simulink model "sogi_discrete_comparison"  (R2026a)
settings: Solver=FixedStepDiscrete  StopTime=1  FixedStep=double(Cal_SOGI_Ts_s_f32)
PostLoadFcn:
  | addpath(fileparts(get_param('sogi_discrete_comparison','FileName'))); sogi_refresh_parameter_panels('sogi_discrete_comparison');
InitFcn:
  | sogi_check_parameter_binding('sogi_discrete_comparison',false);
StartFcn:
  | sogi_check_parameter_binding('sogi_discrete_comparison',true,true);
values from neighbouring files (symbols this model uses):
  Cal_SOGI_BEA11_f32 = 0.978032291    [sogi_parameters.sldd]
  Cal_SOGI_BEA12_f32 = -0.0153628942    [sogi_parameters.sldd]
  Cal_SOGI_BEA21_f32 = 0.0153628942    [sogi_parameters.sldd]
  Cal_SOGI_BEA22_f32 = 0.999758661    [sogi_parameters.sldd]
  Cal_SOGI_BEB11_f32 = 0.0217264127    [sogi_parameters.sldd]
  Cal_SOGI_BEB21_f32 = 0.000341277686    [sogi_parameters.sldd]
  Cal_SOGI_BEC11_f32 = 0.978032291    [sogi_parameters.sldd]
  Cal_SOGI_BEC12_f32 = -0.0153628942    [sogi_parameters.sldd]
  Cal_SOGI_BEC21_f32 = 0.0153628942    [sogi_parameters.sldd]
  Cal_SOGI_BEC22_f32 = 0.999758661    [sogi_parameters.sldd]
  Cal_SOGI_BED11_f32 = 0.0217264127    [sogi_parameters.sldd]
  Cal_SOGI_BED21_f32 = 0.000341277686    [sogi_parameters.sldd]
  Cal_SOGI_Ts_s_f32 = 5.0E-5    [sogi_parameters.sldd]
  Cal_SOGI_TustinA11_f32 = 0.977908969    [sogi_parameters.sldd]
  Cal_SOGI_TustinA12_f32 = -0.0155344605    [sogi_parameters.sldd]
  Cal_SOGI_TustinA21_f32 = 0.0155344605    [sogi_parameters.sldd]
  Cal_SOGI_TustinA22_f32 = 0.999878    [sogi_parameters.sldd]
  Cal_SOGI_TustinB11_f32 = 0.0219690446    [sogi_parameters.sldd]
  Cal_SOGI_TustinB21_f32 = 0.00017254446    [sogi_parameters.sldd]
  Cal_SOGI_TustinC11_f32 = 0.988954484    [sogi_parameters.sldd]
  Cal_SOGI_TustinC12_f32 = -0.00776723027    [sogi_parameters.sldd]
  Cal_SOGI_TustinC21_f32 = 0.00776723027    [sogi_parameters.sldd]
  Cal_SOGI_TustinC22_f32 = 0.999939    [sogi_parameters.sldd]
  Cal_SOGI_TustinD11_f32 = 0.0109845223    [sogi_parameters.sldd]
  Cal_SOGI_TustinD21_f32 = 8.627223E-5    [sogi_parameters.sldd]
  Cal_SOGI_ZOHA11_f32 = 0.977908969    [sogi_parameters.sldd]
  Cal_SOGI_ZOHA12_f32 = -0.0155341374    [sogi_parameters.sldd]
  Cal_SOGI_ZOHA21_f32 = 0.0155341374    [sogi_parameters.sldd]
  Cal_SOGI_ZOHA22_f32 = 0.999877512    [sogi_parameters.sldd]
  Cal_SOGI_ZOHB11_f32 = 0.0219685864    [sogi_parameters.sldd]
  Cal_SOGI_ZOHB21_f32 = 0.000173183245    [sogi_parameters.sldd]
  Cal_SOGI_ZOHC11_f32 = 1.0    [sogi_parameters.sldd]
  Cal_SOGI_ZOHC12_f32 = 0.0    [sogi_parameters.sldd]
  Cal_SOGI_ZOHC21_f32 = 0.0    [sogi_parameters.sldd]
  Cal_SOGI_ZOHC22_f32 = 1.0    [sogi_parameters.sldd]
  Cal_SOGI_ZOHD11_f32 = 0.0    [sogi_parameters.sldd]
  Cal_SOGI_ZOHD21_f32 = 0.0    [sogi_parameters.sldd]
settings Model: DataDictionary=sogi_parameters.sldd  EnableAccessToBaseWorkspace=off  Creator=ASUS  LastModifiedBy=ASUS

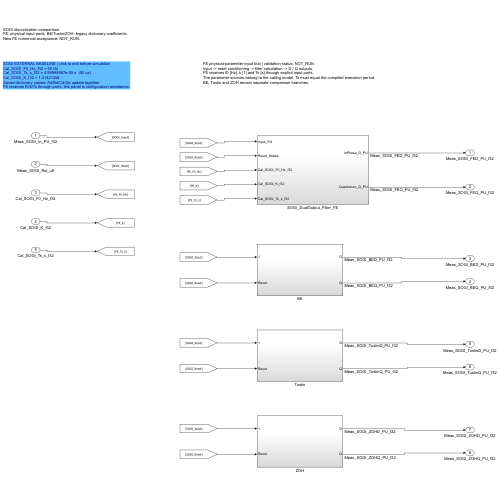
[thumbnail: Simulink's stored preview of the top-level diagram]
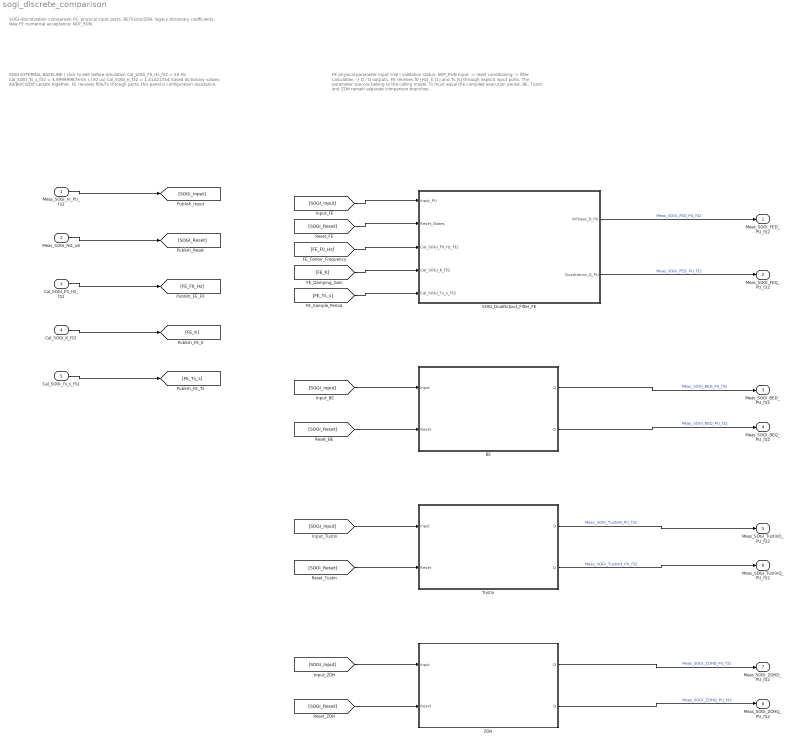
== system sogi_discrete_comparison ==
  note: SOGI discretization comparison
      | FE: physical input ports. BE/Tustin/ZOH: legacy dictionary coefficients.
      | New FE numerical acceptance: NOT_RUN.
  note: SOGI EXTERNAL BASELINE | click to edit before simulation
      | Cal_SOGI_F0_Hz_f32 = 50 Hz
      | Cal_SOGI_Ts_s_f32 = 4.99999987e-05 s  (50 us)
      | Cal_SOGI_K_f32 = 1.41421354
      | Saved dictionary values; Ad/Bd/Cd/Dd update together.
      | FE receives f0/k/Ts through ports; this panel is configuration assistance.
  note: FE physical-parameter input trial | validation status: NOT_RUN
      | Input -> reset conditioning -> filter calculation -> D / Q outputs.
      | FE receives f0 [Hz], k [1] and Ts [s] through explicit input ports.
      | The parameter sources belong to the calling model. Ts must equal the compiled execution period.
      | BE, Tustin and ZOH remain separate comparison branches.
  Meas_SOGI_In_PU_f32 : Inport  OutDataTypeStr=single  SampleTime=double(Cal_SOGI_Ts_s_f32)
  Meas_SOGI_Rst_u8 : Inport  Port=2  OutDataTypeStr=uint8  SampleTime=double(Cal_SOGI_Ts_s_f32)
  Cal_SOGI_F0_Hz_f32 : Inport  Port=3  OutDataTypeStr=single  SampleTime=double(Cal_SOGI_Ts_s_f32)
  Cal_SOGI_K_f32 : Inport  Port=4  OutDataTypeStr=single  SampleTime=double(Cal_SOGI_Ts_s_f32)
  Cal_SOGI_Ts_s_f32 : Inport  Port=5  OutDataTypeStr=single  SampleTime=double(Cal_SOGI_Ts_s_f32)
  BE : Subsystem
  SOGI_DualOutput_Filter_FE : Subsystem  Tag=SOGI_METHOD_FE
  Tustin : Subsystem
  ZOH : Subsystem
  Meas_SOGI_FED_PU_f32 : Outport  OutDataTypeStr=single
  Meas_SOGI_FEQ_PU_f32 : Outport  Port=2  OutDataTypeStr=single
  Meas_SOGI_BED_PU_f32 : Outport  Port=3  OutDataTypeStr=single
  Meas_SOGI_BEQ_PU_f32 : Outport  Port=4  OutDataTypeStr=single
  Meas_SOGI_TustinD_PU_f32 : Outport  Port=5  OutDataTypeStr=single
  Meas_SOGI_TustinQ_PU_f32 : Outport  Port=6  OutDataTypeStr=single
  Meas_SOGI_ZOHD_PU_f32 : Outport  Port=7  OutDataTypeStr=single
  Meas_SOGI_ZOHQ_PU_f32 : Outport  Port=8  OutDataTypeStr=single
  wires:
  [SOGI_Reset] -> ZOH/2(Reset)
  [SOGI_Input] -> ZOH/1(Input)
  [SOGI_Reset] -> Tustin/2(Reset)
  [SOGI_Input] -> Tustin/1(Input)
  [SOGI_Reset] -> BE/2(Reset)
  [SOGI_Input] -> BE/1(Input)
  [SOGI_Reset] -> SOGI_DualOutput_Filter_FE/2(Reset_States)
  [SOGI_Input] -> SOGI_DualOutput_Filter_FE/1(Input_PU)
  ZOH/2(Q) -> Meas_SOGI_ZOHQ_PU_f32/1  "Meas_SOGI_ZOHQ_PU_f32"
  ZOH/1(D) -> Meas_SOGI_ZOHD_PU_f32/1  "Meas_SOGI_ZOHD_PU_f32"
  Tustin/2(Q) -> Meas_SOGI_TustinQ_PU_f32/1  "Meas_SOGI_TustinQ_PU_f32"
  Tustin/1(D) -> Meas_SOGI_TustinD_PU_f32/1  "Meas_SOGI_TustinD_PU_f32"
  BE/2(Q) -> Meas_SOGI_BEQ_PU_f32/1  "Meas_SOGI_BEQ_PU_f32"
  BE/1(D) -> Meas_SOGI_BED_PU_f32/1  "Meas_SOGI_BED_PU_f32"
  SOGI_DualOutput_Filter_FE/2(Quadrature_Q_PU) -> Meas_SOGI_FEQ_PU_f32/1  "Meas_SOGI_FEQ_PU_f32"
  SOGI_DualOutput_Filter_FE/1(InPhase_D_PU) -> Meas_SOGI_FED_PU_f32/1  "Meas_SOGI_FED_PU_f32"
  Meas_SOGI_Rst_u8/1 -> [SOGI_Reset]
  Meas_SOGI_In_PU_f32/1 -> [SOGI_Input]
  [FE_Ts_s] -> SOGI_DualOutput_Filter_FE/5(Cal_SOGI_Ts_s_f32)
  [FE_K] -> SOGI_DualOutput_Filter_FE/4(Cal_SOGI_K_f32)
  [FE_F0_Hz] -> SOGI_DualOutput_Filter_FE/3(Cal_SOGI_F0_Hz_f32)
  Cal_SOGI_Ts_s_f32/1 -> [FE_Ts_s]
  Cal_SOGI_K_f32/1 -> [FE_K]
  Cal_SOGI_F0_Hz_f32/1 -> [FE_F0_Hz]

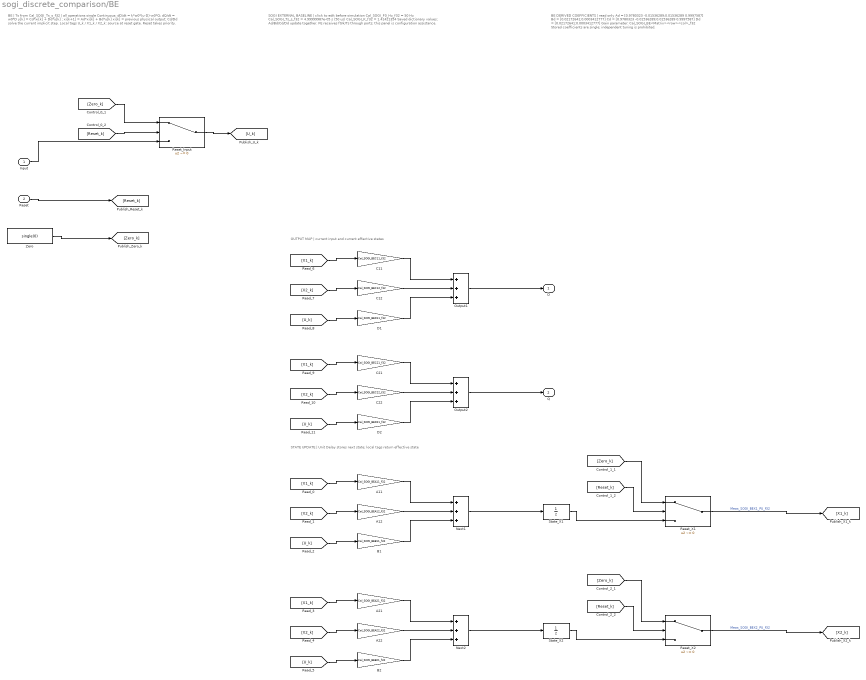
== system sogi_discrete_comparison/BE ==
  note: BE | Ts from Cal_SOGI_Ts_s_f32 | all operations single
      | Continuous: dD/dt = k*w0*(u-D)-w0*Q; dQ/dt = w0*D
      | y[k] = Cd*xi[k] + Dd*u[k]   ;   xi[k+1] = Ad*xi[k] + Bd*u[k]
      | xi[k] = previous physical output; Cd/Dd solve the current implicit step.
      | Local tags U_k / X1_k / X2_k: source at reset gate. Reset takes priority.
  note: OUTPUT MAP | current input and current effective states
  note: STATE UPDATE | Unit Delay stores next state; local tags return effective state
  note: SOGI EXTERNAL BASELINE | click to edit before simulation
      | Cal_SOGI_F0_Hz_f32 = 50 Hz
      | Cal_SOGI_Ts_s_f32 = 4.99999987e-05 s  (50 us)
      | Cal_SOGI_K_f32 = 1.41421354
      | Saved dictionary values; Ad/Bd/Cd/Dd update together.
      | FE receives f0/k/Ts through ports; this panel is configuration assistance.
  note: BE DERIVED COEFFICIENTS | read only
      | Ad = [0.9780323 -0.01536289;0.01536289 0.9997587]
      | Bd = [0.02172641;0.0003412777]
      | Cd = [0.9780323 -0.01536289;0.01536289 0.9997587]
      | Dd = [0.02172641;0.0003412777]
      | Gain parameter: Cal_SOGI_BE<Matrix><row><col>_f32
      | Stored coefficients are single; independent tuning is prohibited.
  Input : Inport
  Reset : Inport  Port=2
  A11 : Gain  Gain=Cal_SOGI_BEA11_f32  ParamDataTypeStr=single  OutDataTypeStr=single
  A12 : Gain  Gain=Cal_SOGI_BEA12_f32  ParamDataTypeStr=single  OutDataTypeStr=single
  A21 : Gain  Gain=Cal_SOGI_BEA21_f32  ParamDataTypeStr=single  OutDataTypeStr=single
  A22 : Gain  Gain=Cal_SOGI_BEA22_f32  ParamDataTypeStr=single  OutDataTypeStr=single
  B1 : Gain  Gain=Cal_SOGI_BEB11_f32  ParamDataTypeStr=single  OutDataTypeStr=single
  B2 : Gain  Gain=Cal_SOGI_BEB21_f32  ParamDataTypeStr=single  OutDataTypeStr=single
  C11 : Gain  Gain=Cal_SOGI_BEC11_f32  ParamDataTypeStr=single  OutDataTypeStr=single
  C12 : Gain  Gain=Cal_SOGI_BEC12_f32  ParamDataTypeStr=single  OutDataTypeStr=single
  C21 : Gain  Gain=Cal_SOGI_BEC21_f32  ParamDataTypeStr=single  OutDataTypeStr=single
  C22 : Gain  Gain=Cal_SOGI_BEC22_f32  ParamDataTypeStr=single  OutDataTypeStr=single
  D1 : Gain  Gain=Cal_SOGI_BED11_f32  ParamDataTypeStr=single  OutDataTypeStr=single
  D2 : Gain  Gain=Cal_SOGI_BED21_f32  ParamDataTypeStr=single  OutDataTypeStr=single
  Next1 : Sum  Inputs=+++  OutDataTypeStr=single  AccumDataTypeStr=single
  Next2 : Sum  Inputs=+++  OutDataTypeStr=single  AccumDataTypeStr=single
  Output1 : Sum  Inputs=+++  OutDataTypeStr=single  AccumDataTypeStr=single
  Output2 : Sum  Inputs=+++  OutDataTypeStr=single  AccumDataTypeStr=single
  Reset_Input : Switch  Criteria=u2 ~= 0  OutDataTypeStr=single  SaturateOnIntegerOverflow=off  InputSameDT=off
  Reset_X1 : Switch  Criteria=u2 ~= 0  OutDataTypeStr=single  SaturateOnIntegerOverflow=off  InputSameDT=off
  Reset_X2 : Switch  Criteria=u2 ~= 0  OutDataTypeStr=single  SaturateOnIntegerOverflow=off  InputSameDT=off
  State_X1 : UnitDelay  InitialCondition=single(0)  SampleTime=double(Cal_SOGI_Ts_s_f32)
  State_X2 : UnitDelay  InitialCondition=single(0)  SampleTime=double(Cal_SOGI_Ts_s_f32)
  Zero : Constant  Value=single(0)  OutDataTypeStr=single
  D : Outport
  Q : Outport  Port=2
  wires:
  Reset/1 -> [Reset_k]
  [Reset_k] -> Reset_X2/2
  [Zero_k] -> Reset_X2/1
  [Reset_k] -> Reset_X1/2
  [Zero_k] -> Reset_X1/1
  [Reset_k] -> Reset_Input/2
  [Zero_k] -> Reset_Input/1
  [U_k] -> D2/1
  [X2_k] -> C22/1
  [X1_k] -> C21/1
  [U_k] -> D1/1
  [X2_k] -> C12/1
  [X1_k] -> C11/1
  [U_k] -> B2/1
  [X2_k] -> A22/1
  [X1_k] -> A21/1
  [U_k] -> B1/1
  [X2_k] -> A12/1
  [X1_k] -> A11/1
  Output2/1 -> Q/1
  D2/1 -> Output2/3
  C22/1 -> Output2/2
  C21/1 -> Output2/1
  Output1/1 -> D/1
  D1/1 -> Output1/3
  C12/1 -> Output1/2
  C11/1 -> Output1/1
  Next2/1 -> State_X2/1
  B2/1 -> Next2/3
  A22/1 -> Next2/2
  A21/1 -> Next2/1
  Next1/1 -> State_X1/1
  B1/1 -> Next1/3
  Reset_Input/1 -> [U_k]
  A12/1 -> Next1/2
  Reset_X2/1 -> [X2_k]  "Meas_SOGI_BEX2_PU_f32"
  A11/1 -> Next1/1
  Reset_X1/1 -> [X1_k]  "Meas_SOGI_BEX1_PU_f32"
  State_X2/1 -> Reset_X2/3
  State_X1/1 -> Reset_X1/3
  Zero/1 -> [Zero_k]
  Input/1 -> Reset_Input/3

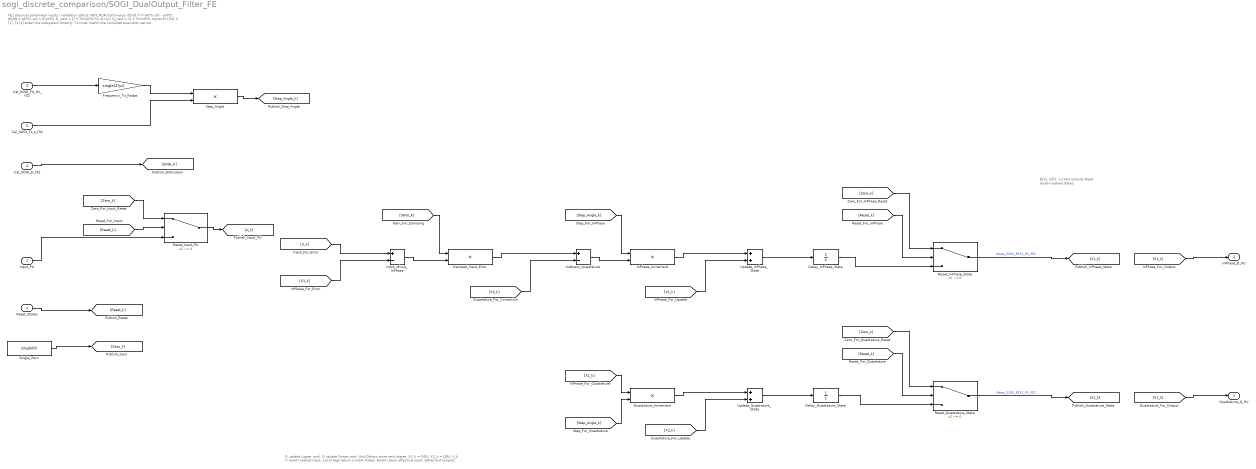
== system sogi_discrete_comparison/SOGI_DualOutput_Filter_FE ==
  note: FE | physical parameter inputs | validation status: NOT_RUN
      | Continuous: dD/dt = k*w0*(u-D) - w0*Q; dQ/dt = w0*D; w0 = 2*pi*f0.
      | D_next = D + Ts*w0*(k*(u-D)-Q); Q_next = Q + Ts*w0*D.
      | Inputs f0 [Hz], k [1], Ts [s] enter this subsystem directly. Ts must match the compiled execution period.
  note: D[k], Q[k]: current outputs
      | Read reset-masked states.
  note: D update (upper row), Q update (lower row); Unit Delays store next states.
      | X1_k = D[k]; X2_k = Q[k]; U_k = reset-masked input.
      | Local tags return current states. Reset clears effective input, states and outputs.
  Input_PU : Inport
  Reset_States : Inport  Port=2
  Cal_SOGI_F0_Hz_f32 : Inport  Port=3  OutDataTypeStr=single
  Cal_SOGI_K_f32 : Inport  Port=4  OutDataTypeStr=single
  Cal_SOGI_Ts_s_f32 : Inport  Port=5  OutDataTypeStr=single
  Damped_Input_Error : Product  Inputs=**  OutDataTypeStr=single
  Delay_InPhase_State : UnitDelay  InitialCondition=single(0)  SampleTime=-1
  Delay_Quadrature_State : UnitDelay  InitialCondition=single(0)  SampleTime=-1
  Frequency_To_Radps : Gain  Gain=single(2*pi)  OutDataTypeStr=single
  InPhase_Increment : Product  Inputs=**  OutDataTypeStr=single
  Input_Minus_InPhase : Sum  Inputs=+-  OutDataTypeStr=single
  Quadrature_Increment : Product  Inputs=**  OutDataTypeStr=single
  Reset_InPhase_State : Switch  Criteria=u2 ~= 0  OutDataTypeStr=single  SaturateOnIntegerOverflow=off  InputSameDT=off
  Reset_Input_PU : Switch  Criteria=u2 ~= 0  OutDataTypeStr=single  SaturateOnIntegerOverflow=off  InputSameDT=off
  Reset_Quadrature_State : Switch  Criteria=u2 ~= 0  OutDataTypeStr=single  SaturateOnIntegerOverflow=off  InputSameDT=off
  Single_Zero : Constant  Value=single(0)  OutDataTypeStr=single
  Step_Angle : Product  Inputs=**  OutDataTypeStr=single
  Subtract_Quadrature : Sum  Inputs=+-  OutDataTypeStr=single
  Update_InPhase_State : Sum  OutDataTypeStr=single
  Update_Quadrature_State : Sum  OutDataTypeStr=single
  InPhase_D_PU : Outport
  Quadrature_Q_PU : Outport  Port=2
  wires:
  Reset_States/1 -> [Reset_k]
  Input_PU/1 -> Reset_Input_PU/3
  [Reset_k] -> Reset_Quadrature_State/2
  [Zero_k] -> Reset_Quadrature_State/1
  [Reset_k] -> Reset_InPhase_State/2
  [Zero_k] -> Reset_InPhase_State/1
  [Reset_k] -> Reset_Input_PU/2
  [Zero_k] -> Reset_Input_PU/1
  Reset_Input_PU/1 -> [U_k]
  Reset_Quadrature_State/1 -> [X2_k]  "Meas_SOGI_FEX2_PU_f32"
  Reset_InPhase_State/1 -> [X1_k]  "Meas_SOGI_FEX1_PU_f32"
  Single_Zero/1 -> [Zero_k]
  Update_Quadrature_State/1 -> Delay_Quadrature_State/1
  [X2_k] -> Update_Quadrature_State/2
  Quadrature_Increment/1 -> Update_Quadrature_State/1
  [Step_Angle_k] -> Quadrature_Increment/2
  [X1_k] -> Quadrature_Increment/1
  Update_InPhase_State/1 -> Delay_InPhase_State/1
  [X1_k] -> Update_InPhase_State/2
  Delay_InPhase_State/1 -> Reset_InPhase_State/3
  Delay_Quadrature_State/1 -> Reset_Quadrature_State/3
  Cal_SOGI_Ts_s_f32/1 -> Step_Angle/2
  Step_Angle/1 -> [Step_Angle_k]
  Cal_SOGI_K_f32/1 -> [SOGI_K]
  [X2_k] -> Quadrature_Q_PU/1
  [X1_k] -> InPhase_D_PU/1
  Frequency_To_Radps/1 -> Step_Angle/1
  Cal_SOGI_F0_Hz_f32/1 -> Frequency_To_Radps/1
  Subtract_Quadrature/1 -> InPhase_Increment/2
  [Step_Angle_k] -> InPhase_Increment/1
  Input_Minus_InPhase/1 -> Damped_Input_Error/2
  [SOGI_K] -> Damped_Input_Error/1
  [U_k] -> Input_Minus_InPhase/1
  [X1_k] -> Input_Minus_InPhase/2
  Damped_Input_Error/1 -> Subtract_Quadrature/1
  [X2_k] -> Subtract_Quadrature/2
  InPhase_Increment/1 -> Update_InPhase_State/1

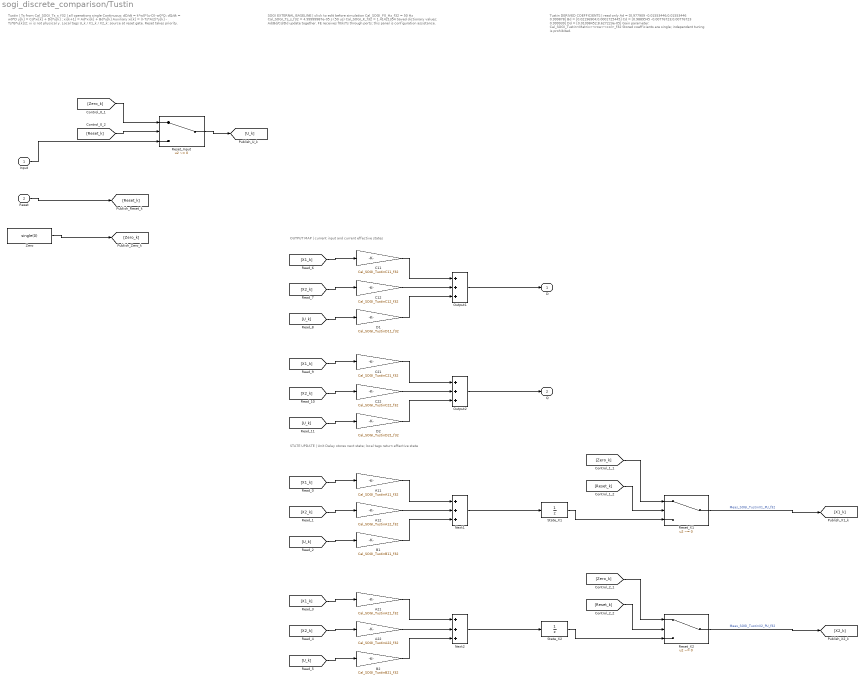
== system sogi_discrete_comparison/Tustin ==
  note: Tustin | Ts from Cal_SOGI_Ts_s_f32 | all operations single
      | Continuous: dD/dt = k*w0*(u-D)-w0*Q; dQ/dt = w0*D
      | y[k] = Cd*xi[k] + Dd*u[k]   ;   xi[k+1] = Ad*xi[k] + Bd*u[k]
      | Auxiliary xi[k] = (I-Ts*A/2)*y[k] - Ts*B*u[k]/2; xi is not physical y.
      | Local tags U_k / X1_k / X2_k: source at reset gate. Reset takes priority.
  note: OUTPUT MAP | current input and current effective states
  note: STATE UPDATE | Unit Delay stores next state; local tags return effective state
  note: SOGI EXTERNAL BASELINE | click to edit before simulation
      | Cal_SOGI_F0_Hz_f32 = 50 Hz
      | Cal_SOGI_Ts_s_f32 = 4.99999987e-05 s  (50 us)
      | Cal_SOGI_K_f32 = 1.41421354
      | Saved dictionary values; Ad/Bd/Cd/Dd update together.
      | FE receives f0/k/Ts through ports; this panel is configuration assistance.
  note: Tustin DERIVED COEFFICIENTS | read only
      | Ad = [0.977909 -0.01553446;0.01553446 0.999878]
      | Bd = [0.02196904;0.0001725445]
      | Cd = [0.9889545 -0.00776723;0.00776723 0.999939]
      | Dd = [0.01098452;8.627223e-05]
      | Gain parameter: Cal_SOGI_Tustin<Matrix><row><col>_f32
      | Stored coefficients are single; independent tuning is prohibited.
  Input : Inport
  Reset : Inport  Port=2
  A11 : Gain  Gain=Cal_SOGI_TustinA11_f32  ParamDataTypeStr=single  OutDataTypeStr=single
  A12 : Gain  Gain=Cal_SOGI_TustinA12_f32  ParamDataTypeStr=single  OutDataTypeStr=single
  A21 : Gain  Gain=Cal_SOGI_TustinA21_f32  ParamDataTypeStr=single  OutDataTypeStr=single
  A22 : Gain  Gain=Cal_SOGI_TustinA22_f32  ParamDataTypeStr=single  OutDataTypeStr=single
  B1 : Gain  Gain=Cal_SOGI_TustinB11_f32  ParamDataTypeStr=single  OutDataTypeStr=single
  B2 : Gain  Gain=Cal_SOGI_TustinB21_f32  ParamDataTypeStr=single  OutDataTypeStr=single
  C11 : Gain  Gain=Cal_SOGI_TustinC11_f32  ParamDataTypeStr=single  OutDataTypeStr=single
  C12 : Gain  Gain=Cal_SOGI_TustinC12_f32  ParamDataTypeStr=single  OutDataTypeStr=single
  C21 : Gain  Gain=Cal_SOGI_TustinC21_f32  ParamDataTypeStr=single  OutDataTypeStr=single
  C22 : Gain  Gain=Cal_SOGI_TustinC22_f32  ParamDataTypeStr=single  OutDataTypeStr=single
  D1 : Gain  Gain=Cal_SOGI_TustinD11_f32  ParamDataTypeStr=single  OutDataTypeStr=single
  D2 : Gain  Gain=Cal_SOGI_TustinD21_f32  ParamDataTypeStr=single  OutDataTypeStr=single
  Next1 : Sum  Inputs=+++  OutDataTypeStr=single  AccumDataTypeStr=single
  Next2 : Sum  Inputs=+++  OutDataTypeStr=single  AccumDataTypeStr=single
  Output1 : Sum  Inputs=+++  OutDataTypeStr=single  AccumDataTypeStr=single
  Output2 : Sum  Inputs=+++  OutDataTypeStr=single  AccumDataTypeStr=single
  Reset_Input : Switch  Criteria=u2 ~= 0  OutDataTypeStr=single  SaturateOnIntegerOverflow=off  InputSameDT=off
  Reset_X1 : Switch  Criteria=u2 ~= 0  OutDataTypeStr=single  SaturateOnIntegerOverflow=off  InputSameDT=off
  Reset_X2 : Switch  Criteria=u2 ~= 0  OutDataTypeStr=single  SaturateOnIntegerOverflow=off  InputSameDT=off
  State_X1 : UnitDelay  InitialCondition=single(0)  SampleTime=double(Cal_SOGI_Ts_s_f32)
  State_X2 : UnitDelay  InitialCondition=single(0)  SampleTime=double(Cal_SOGI_Ts_s_f32)
  Zero : Constant  Value=single(0)  OutDataTypeStr=single
  D : Outport
  Q : Outport  Port=2
  wires:
  Reset/1 -> [Reset_k]
  [Reset_k] -> Reset_X2/2
  [Zero_k] -> Reset_X2/1
  [Reset_k] -> Reset_X1/2
  [Zero_k] -> Reset_X1/1
  [Zero_k] -> Reset_Input/1
  [U_k] -> D2/1
  [X2_k] -> C22/1
  [X1_k] -> C21/1
  [U_k] -> D1/1
  [X2_k] -> C12/1
  [X1_k] -> C11/1
  [U_k] -> B2/1
  [X2_k] -> A22/1
  [X1_k] -> A21/1
  [U_k] -> B1/1
  [X2_k] -> A12/1
  [X1_k] -> A11/1
  Output2/1 -> Q/1
  D2/1 -> Output2/3
  C22/1 -> Output2/2
  C21/1 -> Output2/1
  Output1/1 -> D/1
  D1/1 -> Output1/3
  C12/1 -> Output1/2
  C11/1 -> Output1/1
  Next2/1 -> State_X2/1
  B2/1 -> Next2/3
  A22/1 -> Next2/2
  A21/1 -> Next2/1
  Next1/1 -> State_X1/1
  B1/1 -> Next1/3
  Reset_Input/1 -> [U_k]
  A12/1 -> Next1/2
  Reset_X2/1 -> [X2_k]  "Meas_SOGI_TustinX2_PU_f32"
  A11/1 -> Next1/1
  Reset_X1/1 -> [X1_k]  "Meas_SOGI_TustinX1_PU_f32"
  State_X2/1 -> Reset_X2/3
  State_X1/1 -> Reset_X1/3
  Zero/1 -> [Zero_k]
  Input/1 -> Reset_Input/3
  [Reset_k] -> Reset_Input/2

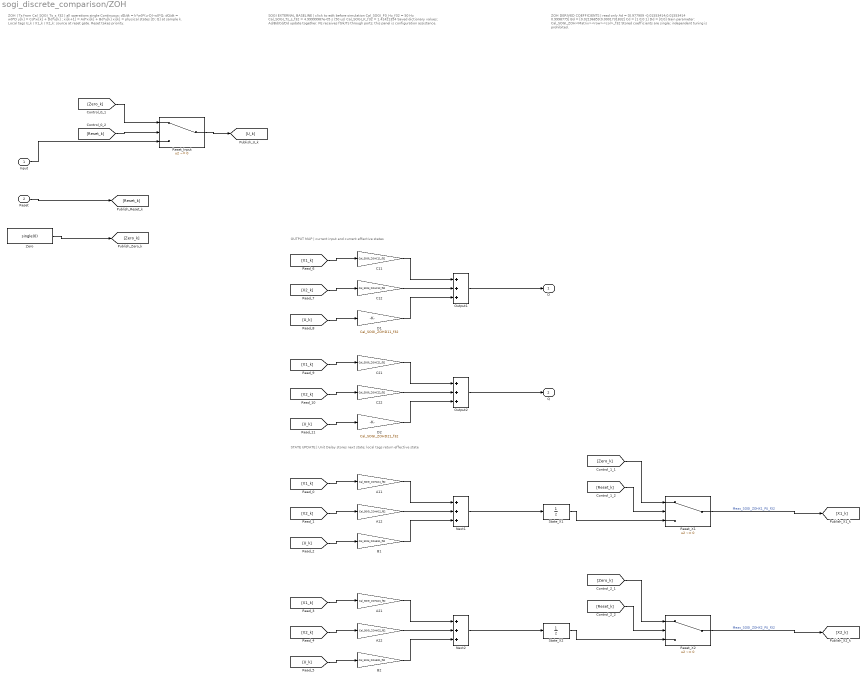
== system sogi_discrete_comparison/ZOH ==
  note: ZOH | Ts from Cal_SOGI_Ts_s_f32 | all operations single
      | Continuous: dD/dt = k*w0*(u-D)-w0*Q; dQ/dt = w0*D
      | y[k] = Cd*xi[k] + Dd*u[k]   ;   xi[k+1] = Ad*xi[k] + Bd*u[k]
      | xi[k] = physical states [D; Q] at sample k.
      | Local tags U_k / X1_k / X2_k: source at reset gate. Reset takes priority.
  note: OUTPUT MAP | current input and current effective states
  note: STATE UPDATE | Unit Delay stores next state; local tags return effective state
  note: SOGI EXTERNAL BASELINE | click to edit before simulation
      | Cal_SOGI_F0_Hz_f32 = 50 Hz
      | Cal_SOGI_Ts_s_f32 = 4.99999987e-05 s  (50 us)
      | Cal_SOGI_K_f32 = 1.41421354
      | Saved dictionary values; Ad/Bd/Cd/Dd update together.
      | FE receives f0/k/Ts through ports; this panel is configuration assistance.
  note: ZOH DERIVED COEFFICIENTS | read only
      | Ad = [0.977909 -0.01553414;0.01553414 0.9998775]
      | Bd = [0.02196859;0.0001731832]
      | Cd = [1 0;0 1]
      | Dd = [0;0]
      | Gain parameter: Cal_SOGI_ZOH<Matrix><row><col>_f32
      | Stored coefficients are single; independent tuning is prohibited.
  Input : Inport
  Reset : Inport  Port=2
  A11 : Gain  Gain=Cal_SOGI_ZOHA11_f32  ParamDataTypeStr=single  OutDataTypeStr=single
  A12 : Gain  Gain=Cal_SOGI_ZOHA12_f32  ParamDataTypeStr=single  OutDataTypeStr=single
  A21 : Gain  Gain=Cal_SOGI_ZOHA21_f32  ParamDataTypeStr=single  OutDataTypeStr=single
  A22 : Gain  Gain=Cal_SOGI_ZOHA22_f32  ParamDataTypeStr=single  OutDataTypeStr=single
  B1 : Gain  Gain=Cal_SOGI_ZOHB11_f32  ParamDataTypeStr=single  OutDataTypeStr=single
  B2 : Gain  Gain=Cal_SOGI_ZOHB21_f32  ParamDataTypeStr=single  OutDataTypeStr=single
  C11 : Gain  Gain=Cal_SOGI_ZOHC11_f32  ParamDataTypeStr=single  OutDataTypeStr=single
  C12 : Gain  Gain=Cal_SOGI_ZOHC12_f32  ParamDataTypeStr=single  OutDataTypeStr=single
  C21 : Gain  Gain=Cal_SOGI_ZOHC21_f32  ParamDataTypeStr=single  OutDataTypeStr=single
  C22 : Gain  Gain=Cal_SOGI_ZOHC22_f32  ParamDataTypeStr=single  OutDataTypeStr=single
  D1 : Gain  Gain=Cal_SOGI_ZOHD11_f32  ParamDataTypeStr=single  OutDataTypeStr=single
  D2 : Gain  Gain=Cal_SOGI_ZOHD21_f32  ParamDataTypeStr=single  OutDataTypeStr=single
  Next1 : Sum  Inputs=+++  OutDataTypeStr=single  AccumDataTypeStr=single
  Next2 : Sum  Inputs=+++  OutDataTypeStr=single  AccumDataTypeStr=single
  Output1 : Sum  Inputs=+++  OutDataTypeStr=single  AccumDataTypeStr=single
  Output2 : Sum  Inputs=+++  OutDataTypeStr=single  AccumDataTypeStr=single
  Reset_Input : Switch  Criteria=u2 ~= 0  OutDataTypeStr=single  SaturateOnIntegerOverflow=off  InputSameDT=off
  Reset_X1 : Switch  Criteria=u2 ~= 0  OutDataTypeStr=single  SaturateOnIntegerOverflow=off  InputSameDT=off
  Reset_X2 : Switch  Criteria=u2 ~= 0  OutDataTypeStr=single  SaturateOnIntegerOverflow=off  InputSameDT=off
  State_X1 : UnitDelay  InitialCondition=single(0)  SampleTime=double(Cal_SOGI_Ts_s_f32)
  State_X2 : UnitDelay  InitialCondition=single(0)  SampleTime=double(Cal_SOGI_Ts_s_f32)
  Zero : Constant  Value=single(0)  OutDataTypeStr=single
  D : Outport
  Q : Outport  Port=2
  wires:
  Reset/1 -> [Reset_k]
  [Reset_k] -> Reset_X2/2
  [Zero_k] -> Reset_X2/1
  [Reset_k] -> Reset_X1/2
  [Zero_k] -> Reset_X1/1
  [Zero_k] -> Reset_Input/1
  [U_k] -> D2/1
  [X2_k] -> C22/1
  [X1_k] -> C21/1
  [U_k] -> D1/1
  [X2_k] -> C12/1
  [X1_k] -> C11/1
  [U_k] -> B2/1
  [X2_k] -> A22/1
  [X1_k] -> A21/1
  [U_k] -> B1/1
  [X2_k] -> A12/1
  [X1_k] -> A11/1
  Output2/1 -> Q/1
  D2/1 -> Output2/3
  C22/1 -> Output2/2
  C21/1 -> Output2/1
  Output1/1 -> D/1
  D1/1 -> Output1/3
  C12/1 -> Output1/2
  C11/1 -> Output1/1
  Next2/1 -> State_X2/1
  B2/1 -> Next2/3
  A22/1 -> Next2/2
  A21/1 -> Next2/1
  Next1/1 -> State_X1/1
  B1/1 -> Next1/3
  Reset_Input/1 -> [U_k]
  A12/1 -> Next1/2
  Reset_X2/1 -> [X2_k]  "Meas_SOGI_ZOHX2_PU_f32"
  A11/1 -> Next1/1
  Reset_X1/1 -> [X1_k]  "Meas_SOGI_ZOHX1_PU_f32"
  State_X2/1 -> Reset_X2/3
  State_X1/1 -> Reset_X1/3
  Zero/1 -> [Zero_k]
  Input/1 -> Reset_Input/3
  [Reset_k] -> Reset_Input/2
